simulink model "fuzzy_projekat"  (R2020b)
settings: Solver=FixedStepAuto  StartTime=0.0  StopTime=1000.0  FixedStep=3  RelTol=1e-3
values from neighbouring files (symbols this model uses):
  KdPD = Kp*Td/KuPD    (= 20.459538)    [fuzzy_matlab.m]
  KdPID = Kp*Td/KuPID    (= 1.8596875)    [fuzzy_matlab.m]
  KiPID = Kp/(Ti*KuPID)    (= 0.00840194925223)    [fuzzy_matlab.m]
  Kkr = 1.146    [fuzzy_matlab.m]
  Kp = 0.6*Kkr    (= 0.6876)    [fuzzy_matlab.m]
  KpP = Kp/KuP    (= 1.3752)    [fuzzy_matlab.m]
  KpPD = Kp/KuPD    (= 2.7504)    [fuzzy_matlab.m]
  KpPID = 0.25    [fuzzy_matlab.m]
  Kuopt = KuPID*0.2    (= 0.55008)    [fuzzy_matlab.m]
  KuP = Umax    (= 0.5)    [fuzzy_matlab.m]
  KuPD = Umax/2    (= 0.25)    [fuzzy_matlab.m]
  KuPID = Kp/KpPID    (= 2.7504)    [fuzzy_matlab.m]
  Td = Tkr/8    (= 7.43875)    [fuzzy_matlab.m]
  Ti = Tkr/2    (= 29.755)    [fuzzy_matlab.m]
libraries: fuzblock x8
settings Model: Creator=Marija  LastModifiedBy=Marija

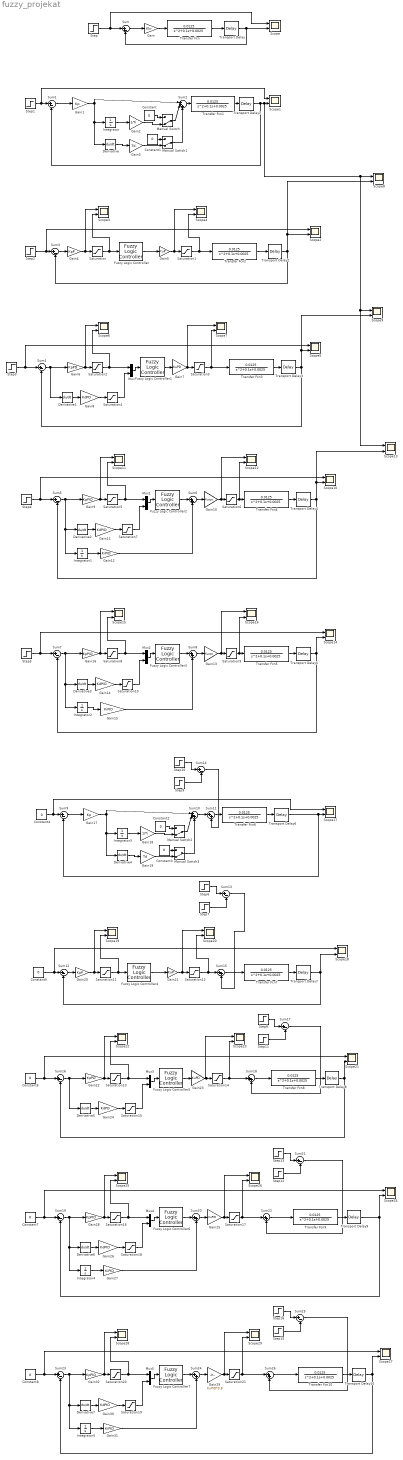
== system fuzzy_projekat ==
  Constant{,1..8} (9 alike) : Constant  Value=0
  Derivative{,1..7} (8 alike) : Derivative
  Fuzzy Logic Controller : fuzblock/Fuzzy Logic  Controller  FIS='P.fis'  OutputSampleNumber=101  DataType=double  FuzzifiedInputs=off  RuleFiringStrengths=off  RuleOutputs=off  AggregatedOutputs=off  SimulateUsing=Interpreted execution  OutOfRangeInputValueMessage=warning  NoRuleFiredMessage=warning  EmptyOutputFuzzySetMessage=warning
  Fuzzy Logic Controller{1..2,5..6} (4 alike) : fuzblock/Fuzzy Logic  Controller  FIS='PD.fis'  OutputSampleNumber=101  DataType=double  FuzzifiedInputs=off  RuleFiringStrengths=off  RuleOutputs=off  AggregatedOutputs=off  SimulateUsing=Interpreted execution  OutOfRangeInputValueMessage=warning  NoRuleFiredMessage=warning  EmptyOutputFuzzySetMessage=warning
  Fuzzy Logic Controller3 : fuzblock/Fuzzy Logic  Controller  FIS='PD_nelinearan.fis'  OutputSampleNumber=101  DataType=double  FuzzifiedInputs=off  RuleFiringStrengths=off  RuleOutputs=off  AggregatedOutputs=off  SimulateUsing=Interpreted execution  OutOfRangeInputValueMessage=warning  NoRuleFiredMessage=warning  EmptyOutputFuzzySetMessage=warning
  Fuzzy Logic Controller4 : fuzblock/Fuzzy Logic  Controller  FIS='P.fis'  OutputSampleNumber=101  DataType=double  FuzzifiedInputs=off  RuleFiringStrengths=off  RuleOutputs=off  AggregatedOutputs=off  SimulateUsing=Interpreted execution  OutOfRangeInputValueMessage=warning  NoRuleFiredMessage=warning  EmptyOutputFuzzySetMessage=warning
  Fuzzy Logic Controller7 : fuzblock/Fuzzy Logic  Controller  FIS='PD_nelinearan.fis'  OutputSampleNumber=101  DataType=double  FuzzifiedInputs=off  RuleFiringStrengths=off  RuleOutputs=off  AggregatedOutputs=off  SimulateUsing=Interpreted execution  OutOfRangeInputValueMessage=warning  NoRuleFiredMessage=warning  EmptyOutputFuzzySetMessage=warning
  Gain : Gain  Gain=Kkr
  Gain1 : Gain  Gain=Kp
  Gain10 : Gain  Gain=Kuopt
  Gain{11,14,26,30} (4 alike) : Gain  Gain=KdPID
  Gain{12,15,27,31} (4 alike) : Gain  Gain=KiPID
  Gain13 : Gain  Gain=Kuopt
  Gain{9,16,28,32} (4 alike) : Gain  Gain=KpPID
  Gain17 : Gain  Gain=Kp
  Gain18 : Gain  Gain=1/Ti
  Gain19 : Gain  Gain=Td
  Gain2 : Gain  Gain=1/Ti
  Gain20 : Gain  Gain=KpP
  Gain21 : Gain  Gain=KuP
  Gain22 : Gain  Gain=KpPD
  Gain23 : Gain  Gain=KuPD
  Gain24 : Gain  Gain=KdPD
  Gain25 : Gain  Gain=KuPID
  Gain29 : Gain  Gain=KuPID*0.8
  Gain3 : Gain  Gain=Td
  Gain4 : Gain  Gain=KpP
  Gain5 : Gain  Gain=KuP
  Gain6 : Gain  Gain=KpPD
  Gain7 : Gain  Gain=KuPD
  Gain8 : Gain  Gain=KdPD
  Integrator{,1..5} (6 alike) : Integrator
  Manual Switch{,1..3} (4 alike) : ManualSwitch  CurrentSetting=0
  Mux{,1..5} (6 alike) : Mux  Inputs=2
  Saturation{,2,4..5,7..8,10..11,13,15..16,18..20} (14 alike) : Saturate  UpperLimit=1  LowerLimit=-1
  Saturation{1,3,6,9,12,14,17,21} (8 alike) : Saturate
  Scope{,1..29} (30 alike) : Scope  NumInputPorts=2
  Step{,1..5} (6 alike) : Step  Time=400  Before=-2  After=2  SampleTime=0
  Step{6,8,10,13,16} (5 alike) : Step  Time=100  After=0.25  SampleTime=0
  Step{7,9,11..12,15} (5 alike) : Step  Time=500  After=0.5  SampleTime=0
  Sum{,1,3..5,7,9,12..14,16..17,19,21,23,25} (16 alike) : Sum  Inputs=|+-
  Sum10 : Sum  Inputs=|+++
  Sum{6,8,11,15,18,20,22,24,26} (9 alike) : Sum  Inputs=|++
  Sum2 : Sum  Inputs=|+++
  Transfer Fcn{,1..10} (11 alike) : TransferFcn  Numerator=[0.0125]  Denominator=[1 0.1 0.0025]
  Transport Delay{,1..10} (11 alike) : TransportDelay  DelayTime=8
  wires:
  Step/1 -> Scope/1, Sum/1
  Gain/1 -> Transfer Fcn/1
  Sum/1 -> Gain/1
  Transfer Fcn/1 -> Transport Delay/1
  Transport Delay/1 -> Scope/2, Sum/2
  Transfer Fcn1/1 -> Transport Delay1/1
  Step1/1 -> Scope1/1, Sum1/1
  Sum2/1 -> Transfer Fcn1/1
  Sum1/1 -> Gain1/1
  Integrator/1 -> Gain2/1
  Derivative/1 -> Gain3/1
  Gain1/1 -> Derivative/1, Integrator/1, Sum2/1
  Transfer Fcn2/1 -> Transport Delay2/1
  Step2/1 -> Sum3/1, Scope2/1
  Sum3/1 -> Gain4/1
  Transport Delay2/1 -> Scope8/2, Scope2/2, Sum3/2
  Saturation1/1 -> Scope4/2, Transfer Fcn2/1
  Gain5/1 -> Scope4/1, Saturation1/1
  Fuzzy Logic Controller/1 -> Gain5/1
  Gain4/1 -> Scope3/1, Saturation/1
  Saturation/1 -> Scope3/2, Fuzzy Logic Controller/1
  Saturation3/1 -> Scope7/2, Transfer Fcn3/1
  Gain6/1 -> Scope6/1, Saturation2/1
  Gain7/1 -> Scope7/1, Saturation3/1
  Fuzzy Logic Controller1/1 -> Gain7/1
  Transfer Fcn3/1 -> Transport Delay3/1
  Sum4/1 -> Derivative1/1, Gain6/1
  Step3/1 -> Sum4/1, Scope5/1
  Transport Delay3/1 -> Scope9/2, Scope5/2, Sum4/2
  Saturation2/1 -> Mux/1, Scope6/2
  Gain2/1 -> Manual Switch/2
  Manual Switch/1 -> Sum2/2
  Constant/1 -> Manual Switch/1
  Mux/1 -> Fuzzy Logic Controller1/1
  Derivative1/1 -> Gain8/1
  Gain8/1 -> Saturation4/1
  Saturation4/1 -> Mux/2
  Transport Delay1/1 -> Scope13/1, Scope9/1, Scope8/1, Scope1/2, Sum1/2
  Manual Switch1/1 -> Sum2/3
  Gain3/1 -> Manual Switch1/2
  Constant1/1 -> Manual Switch1/1
  Saturation7/1 -> Mux1/2
  Mux1/1 -> Fuzzy Logic Controller2/1
  Transport Delay4/1 -> Scope13/2, Scope10/2, Sum5/2
  Step4/1 -> Sum5/1, Scope10/1
  Sum5/1 -> Integrator1/1, Derivative2/1, Gain9/1
  Gain10/1 -> Scope12/1, Saturation6/1
  Gain9/1 -> Scope11/1, Saturation5/1
  Saturation6/1 -> Scope12/2, Transfer Fcn4/1
  Derivative2/1 -> Gain11/1
  Gain11/1 -> Saturation7/1
  Saturation5/1 -> Mux1/1, Scope11/2
  Transfer Fcn4/1 -> Transport Delay4/1
  Sum6/1 -> Gain10/1
  Fuzzy Logic Controller2/1 -> Sum6/1
  Gain12/1 -> Sum6/2
  Integrator1/1 -> Gain12/1
  Transfer Fcn5/1 -> Transport Delay5/1
  Sum8/1 -> Gain13/1
  Integrator2/1 -> Gain15/1
  Gain15/1 -> Sum8/2
  Fuzzy Logic Controller3/1 -> Sum8/1
  Derivative3/1 -> Gain14/1
  Gain14/1 -> Saturation10/1
  Gain16/1 -> Scope15/1, Saturation8/1
  Gain13/1 -> Scope16/1, Saturation9/1
  Sum7/1 -> Integrator2/1, Derivative3/1, Gain16/1
  Step5/1 -> Sum7/1, Scope14/1
  Saturation8/1 -> Mux2/1, Scope15/2
  Mux2/1 -> Fuzzy Logic Controller3/1
  Transport Delay5/1 -> Scope14/2, Sum7/2
  Saturation10/1 -> Mux2/2
  Saturation9/1 -> Scope16/2, Transfer Fcn5/1
  Sum9/1 -> Gain17/1
  Constant4/1 -> Scope17/1, Sum9/1
  Derivative4/1 -> Gain19/1
  Transfer Fcn6/1 -> Transport Delay6/1
  Integrator3/1 -> Gain18/1
  Gain17/1 -> Derivative4/1, Integrator3/1, Sum10/1
  Transport Delay6/1 -> Scope17/2, Sum9/2
  Manual Switch3/1 -> Sum10/3
  Gain19/1 -> Manual Switch3/2
  Gain18/1 -> Manual Switch2/2
  Constant3/1 -> Manual Switch3/1
  Manual Switch2/1 -> Sum10/2
  Constant2/1 -> Manual Switch2/1
  Step10/1 -> Sum14/1
  Step9/1 -> Sum14/2
  Sum11/1 -> Transfer Fcn6/1
  Sum10/1 -> Sum11/1
  Sum14/1 -> Sum11/2
  Transport Delay7/1 -> Scope18/2, Sum12/2
  Sum12/1 -> Gain20/1
  Transfer Fcn7/1 -> Transport Delay7/1
  Saturation12/1 -> Sum15/1, Scope20/2
  Gain21/1 -> Scope20/1, Saturation12/1
  Fuzzy Logic Controller4/1 -> Gain21/1
  Gain20/1 -> Scope19/1, Saturation11/1
  Constant5/1 -> Sum12/1, Scope18/1
  Saturation11/1 -> Scope19/2, Fuzzy Logic Controller4/1
  Step7/1 -> Sum13/2
  Step6/1 -> Sum13/1
  Sum13/1 -> Sum15/2
  Sum15/1 -> Transfer Fcn7/1
  Transport Delay8/1 -> Scope21/2, Sum16/2
  Constant6/1 -> Sum16/1, Scope21/1
  Gain23/1 -> Scope23/1, Saturation14/1
  Gain22/1 -> Scope22/1, Saturation13/1
  Gain24/1 -> Saturation15/1
  Transfer Fcn8/1 -> Transport Delay8/1
  Mux3/1 -> Fuzzy Logic Controller5/1
  Fuzzy Logic Controller5/1 -> Gain23/1
  Derivative5/1 -> Gain24/1
  Saturation15/1 -> Mux3/2
  Saturation14/1 -> Sum18/1, Scope23/2
  Saturation13/1 -> Mux3/1, Scope22/2
  Sum16/1 -> Derivative5/1, Gain22/1
  Step8/1 -> Sum17/1
  Step11/1 -> Sum17/2
  Sum18/1 -> Transfer Fcn8/1
  Sum17/1 -> Sum18/2
  Transport Delay9/1 -> Scope24/2, Sum19/2
  Transfer Fcn9/1 -> Transport Delay9/1
  Gain28/1 -> Scope25/1, Saturation16/1
  Fuzzy Logic Controller6/1 -> Sum20/1
  Mux4/1 -> Fuzzy Logic Controller6/1
  Integrator4/1 -> Gain27/1
  Constant7/1 -> Sum19/1, Scope24/1
  Saturation18/1 -> Mux4/2
  Saturation16/1 -> Mux4/1, Scope25/2
  Gain26/1 -> Saturation18/1
  Gain27/1 -> Sum20/2
  Derivative6/1 -> Gain26/1
  Saturation17/1 -> Sum22/1, Scope26/2
  Gain25/1 -> Scope26/1, Saturation17/1
  Sum20/1 -> Gain25/1
  Sum19/1 -> Integrator4/1, Derivative6/1, Gain28/1
  Step12/1 -> Sum21/2
  Step13/1 -> Sum21/1
  Sum22/1 -> Transfer Fcn9/1
  Sum21/1 -> Sum22/2
  Saturation19/1 -> Mux5/2
  Sum23/1 -> Integrator5/1, Derivative7/1, Gain32/1
  Gain30/1 -> Saturation19/1
  Derivative7/1 -> Gain30/1
  Fuzzy Logic Controller7/1 -> Sum24/1
  Integrator5/1 -> Gain31/1
  Gain29/1 -> Scope29/1, Saturation21/1
  Gain32/1 -> Scope28/1, Saturation20/1
  Constant8/1 -> Sum23/1, Scope27/1
  Transfer Fcn10/1 -> Transport Delay10/1
  Saturation20/1 -> Mux5/1, Scope28/2
  Gain31/1 -> Sum24/2
  Transport Delay10/1 -> Scope27/2, Sum23/2
  Mux5/1 -> Fuzzy Logic Controller7/1
  Saturation21/1 -> Sum26/1, Scope29/2
  Sum24/1 -> Gain29/1
  Step15/1 -> Sum25/2
  Step16/1 -> Sum25/1
  Sum26/1 -> Transfer Fcn10/1
  Sum25/1 -> Sum26/2
